simulink model "vco_phase_noise_3"  (Simulink 7.4)
settings: Solver=ode45  StartTime=0.0  StopTime=.01  MaxStep=.4/(100e6)  RelTol=.25e-3
StopFcn:
  | VCO_plot_dbc_per_hz;
values from neighbouring files (symbols this model uses):
  Fs = OverSample*Freq(end)    [VCO_noise_profile_3.m]
undefined symbols (not defined in the file or in its folder): dBc, dfilt, Hz
libraries: dspstat3 x6, dsparch4 x5, simulink x3, dspbuff3 x3, dspsigops x3, dspsnks4 x3, dspspect3 x1, dspsrcs4 x1
settings Model: Creator=dbenson  LastModifiedBy=Dick
settings OptimizationCC: InlineInvariantSignals=on  InitFltsAndDblsToZero=on
settings DebuggingCC: SaveWithParameterizedLinksMsg=none  SignalResolutionControl=TryResolveAllWithWarning  MultiTaskDSMMsg=warning  MultiTaskCondExecSysMsg=none  Int32ToFloatConvMsg=none  StrictBusMsg=None
settings RTWCC: IncludeERTFirstTime=on
settings GRTTargetCC: TargetFcnLib=ansi_tfl_tmw.mat

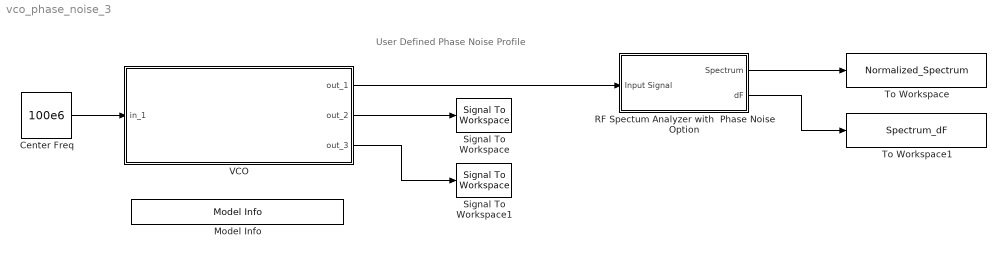
== system vco_phase_noise_3 ==
  note: User Defined Phase Noise Profile
  Center Freq : Constant  Value=100e6  VectorParams1D=off  OutDataType=sfix(16)  OutScaling=2^0
  Model Info : simulink/Model-Wide Utilities/Model Info  SystemSampleTime=-1  InitialBlockCM=None  BlockCM=None  Frame=on  DisplayStringWithTags=Copywrite 2010 The MathWorks, Inc.  HorizontalTextAlignment=Center  LeftAlignmentValue=0.5  SourceBlockDiagram=vco_phase_noise_3  TagMaxNumber=20
  RF Spectum Analyzer with  Phase Noise Option : Subsystem  Description=Spectrum Analyzer  mask{BW=20e6, Fc=100e6, Frame=2^11, Navg=50, N_Toss=2}
      mask prompts: BW "Bandwidth"; Fc "Center Freq"; Frame "Frame Size  (power of 2)"; Navg "Number of Averages"; N_Toss "Toss N Frames b4 Averaging"
      mask Display: fprintf('Spectrum Analyzer \n Fc=%7.2f MHz \n BW=%7.2f MHz',Fc/1e6,BW/1e6)
  Signal To Workspace : dspsnks4/Signal To Workspace  SystemSampleTime=-1  VariableName=Fvec  FrameMode=Concatenate frames (2-D array)
      settings: MaxDataPoints=1  FixptAsFi=off
  Signal To Workspace1 : dspsnks4/Signal To Workspace  SystemSampleTime=-1  VariableName=Lvec  FrameMode=Concatenate frames (2-D array)
      settings: MaxDataPoints=1  FixptAsFi=off
  To Workspace : ToWorkspace  VariableName=Normalized_Spectrum  SampleTime=-1  SaveFormat=Array
      settings: MaxDataPoints=1
  To Workspace1 : ToWorkspace  VariableName=Spectrum_dF  SampleTime=-1  SaveFormat=Array
      settings: MaxDataPoints=1
  VCO : Subsystem  mask{Freq=[ 1e5, 5e5,    2e6,    5e6 ,    8e6   10e6], Level=[-90,   -90,    -100,   -100,    -120 , -120 ]-10, Npts=2^10, OverSample=2.5, Interp_Select=Log X, Ph=0, Kc=1, Fc=0, Ac=sqrt(2)}
      mask prompts: Freq "Phase Noise Freq Vector in Hz"; Level "Phase Noise Level Vector dBc/Hz"; Npts "Phase Noise FIR Filter Length (power of 2)"; OverSample "Phase Noise Oversample (>2)"; Interp_Select "Phase Noise X axis Interpolation"; Ph "Initial Phase (rad)"; Kc "Input Sensitivity (Hz/Volt)"; Fc "Oscillation freq (Hz)"; Ac "Output amplitude (Volt)"
      mask init:
      | Verify=1;
      | noise_filt=VCO_noise_profile_3(Npts,Level,Freq,OverSample,Interp_Select,Verify); 
      | % Npts = length of filter kernel. More provides increased freq resolution
      | % Freq     = Vector of frequencies in Hz
      | % Level = Corresponding Vector of noise levels
      | % Verify   = true to show plots
      | % Create a filter kernel (FIR coefficients) that approximates a user spec'd
      | % power spectrum Level is dB/Hz
      mask StyleString: edit,edit,edit,edit,popup(Linear X|Log X),edit,edit,edit,edit
      mask Display:
      | disp('VCO \nWith User Defined \n Phase Noise (rab)')
      | port_label('input',1','Freq');
      | port_label('output',1','VCO Out');
      | port_label('output',2','Fvec');
      | port_label('output',3','Level');
  wires:
  VCO/1(out_1) -> RF Spectum Analyzer with  Phase Noise Option/1(Input Signal)
  Center Freq/1 -> VCO/1(in_1)
  VCO/2(out_2) -> Signal To Workspace/1
  VCO/3(out_3) -> Signal To Workspace1/1
  RF Spectum Analyzer with  Phase Noise Option/1(Spectrum) -> To Workspace/1
  RF Spectum Analyzer with  Phase Noise Option/2(dF) -> To Workspace1/1

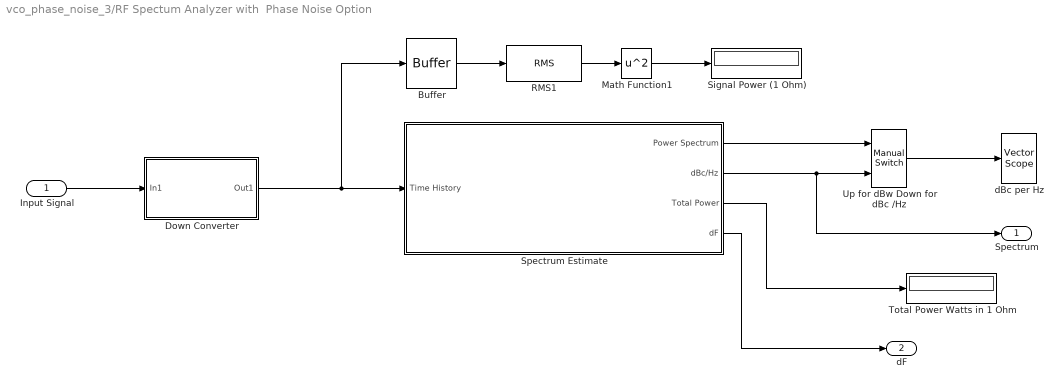
== system vco_phase_noise_3/RF Spectum Analyzer with  Phase Noise Option ==
  Input Signal : Inport  OutDataType=sfix(16)  OutScaling=2^0
  Buffer : dspbuff3/Buffer  N=1024  V=0  ic=0
  Down Converter : Subsystem
  Math Function1 : Math  Operator=square  OutDataType=sfix(16)  OutScaling=2^0  SaturateOnIntegerOverflow=on
  RMS1 : dspstat3/RMS  DialogController=dspDDGCreate  DialogControllerArgs=DataTag0  run=off  reset_popup=None  directionMode=Each column  dimension=1  treatSBRowAsCol=on
  Signal Power (1 Ohm) : Display
  Spectrum Estimate : Subsystem  mask{Frame=Frame, Navg=Navg, N_Toss=N_Toss}
      mask prompts: Frame "Frame Size"; N_Toss "Toos N Frames b4 Averaging"
      mask Display:
      | disp('Power Spectrum \nEstimate')
      | port_label('input',1,'y(t)');
      | port_label('output',1,'Power Spectrum')
      | port_label('output',2,'Scaled for dBc/Hz')
      | port_label('output',3','Total Power');
      | port_label('output',4','dF');
  Total Power Watts in 1 Ohm : Display
  Up for dBw Down for dBc /Hz : simulink/Signal Routing/Manual Switch  SystemSampleTime=-1  sw=0  action=0  varsize=off
  dBc per Hz : dspsnks4/Vector Scope  DialogController=dspdialog.VectorScope  DialogControllerArgs=DataTag5  ScopeProperties=on  Domain=Frequency  HorizSpan=1  DisplayProperties=off  AxisGrid=on  Memory=off  FrameNumber=on  AxisLegend=off  AxisZoom=off  OpenScopeAtSimStart=on  OpenScopeImmediately=off  FigPos=[586 199 560 252]  AxisProperties=off  XUnits=Hertz  XRange=[-Fs/2...Fs/2]  InheritXIncr=on  XIncr=1  XLabel=Time  XLimit=Auto  XMin=0  XMax=1  XStart=0  YUnits=dB  YLabel=dBc/Hz  LineProperties=off  XAxisParamsVer=6.9
      settings: YMin=-164.362362670898  YMax=2.17442076291263e-006
  Spectrum : Outport  OutDataType=fixdt(1, 16)  OutScaling=2^0
  dF : Outport  Port=2  OutDataType=fixdt(1, 16)  OutScaling=2^0
  wires:
  Up for dBw Down for dBc /Hz/1 -> dBc per Hz/1
  Spectrum Estimate/3(Total Power) -> Total Power Watts in 1 Ohm/1
  Spectrum Estimate/2(dBc/Hz) -> Up for dBw Down for dBc /Hz/2, Spectrum/1
  Spectrum Estimate/1(Power Spectrum) -> Up for dBw Down for dBc /Hz/1
  RMS1/1 -> Math Function1/1
  Buffer/1 -> RMS1/1
  Math Function1/1 -> Signal Power (1 Ohm)/1
  Input Signal/1 -> Down Converter/1(In1)
  Down Converter/1(Out1) -> Spectrum Estimate/1(Time History), Buffer/1
  Spectrum Estimate/4(dF) -> dF/1

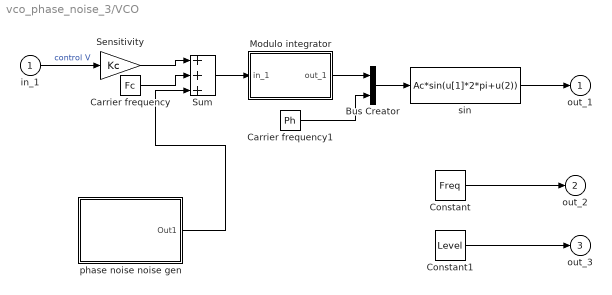
== system vco_phase_noise_3/VCO ==
  in_1 : Inport  OutDataType=sfix(16)  OutScaling=2^0
  Bus Creator : BusCreator  Inputs=2
  Carrier frequency : Constant  Value=Fc  OutDataType=sfix(16)  OutScaling=2^0
  Carrier frequency1 : Constant  Value=Ph  OutDataType=sfix(16)  OutScaling=2^0
  Constant : Constant  Value=Freq  OutDataType=fixdt(1, 16)  OutScaling=2^0
  Constant1 : Constant  Value=Level  OutDataType=fixdt(1, 16)  OutScaling=2^0
  Modulo integrator : Subsystem  mask(Modulo integrator){modu=1, init=0}
      mask prompts: modu "Modulo bound:"; init "Initial state:"
      mask help: When the absolute value of the state exceeds the modulo bound, the state is reset to be the remainder of the state divided by the modulo bound.
      mask Help: This block calculate the integration of the input signal. The absolute value of this integrator will not exceed the specified module bound. The state value is reset to be the remainder of the state divided by the modulo bound. This block can only be used for scale value calculation. This block is a continuous-time integration block.
      mask Display: disp('Modulo\nintegrator')
  Sensitivity : Gain  Gain=Kc  ParameterDataType=sfix(16)  ParameterScaling=2^0  OutDataType=sfix(16)  OutScaling=2^0  SaturateOnIntegerOverflow=on  OutDataTypeStr=Inherit: Same as input  ParamDataTypeStr=Inherit: Same as input
  Sum : Sum  Inputs=+++  OutDataType=sfix(16)  OutScaling=2^0  SaturateOnIntegerOverflow=on  InputSameDT=on  OutDataTypeStr=Inherit: Same as first input
  phase noise noise gen : Subsystem  TreatAsAtomicUnit=on
  sin : Fcn  Expr=Ac*sin(u[1]*2*pi+u(2))
  out_1 : Outport  OutDataType=sfix(16)  OutScaling=2^0
  out_2 : Outport  Port=2  OutDataType=sfix(16)  OutScaling=2^0
  out_3 : Outport  Port=3  OutDataType=sfix(16)  OutScaling=2^0
  wires:
  Modulo integrator/1(out_1) -> Bus Creator/1
  Bus Creator/1 -> sin/1
  Sum/1 -> Modulo integrator/1(in_1)
  sin/1 -> out_1/1
  Carrier frequency/1 -> Sum/2
  Sensitivity/1 -> Sum/1
  in_1/1 -> Sensitivity/1  "control V"
  phase noise noise gen/1(Out1) -> Sum/3
  Constant/1 -> out_2/1
  Constant1/1 -> out_3/1
  Carrier frequency1/1 -> Bus Creator/2

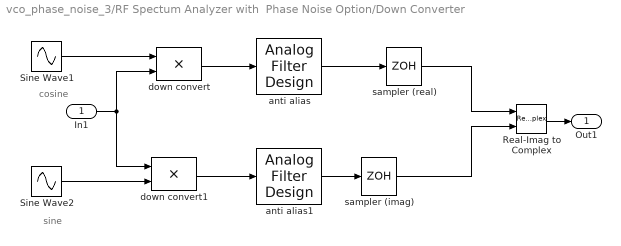
== system vco_phase_noise_3/RF Spectum Analyzer with  Phase Noise Option/Down Converter ==
  note: cosine
  note: sine
  In1 : Inport
  Real-Imag to Complex : RealImagToComplex
  Sine Wave1 : Sin  Amplitude=sqrt(2)  Bias=0  Frequency=2*pi*(Fc)  Phase=-pi/2  Samples=10  SampleTime=0  Offset=0
  Sine Wave2 : Sin  Amplitude=sqrt(2)  Bias=0  Frequency=2*pi*(Fc)  Phase=0  Samples=10  SampleTime=0  Offset=0
  anti alias : dsparch4/Analog Filter Design  method=Elliptic  filttype=Lowpass  N=9  Wlo=BW*pi  Whi=80  Rp=1.2  Rs=100
  anti alias1 : dsparch4/Analog Filter Design  method=Elliptic  filttype=Lowpass  N=9  Wlo=BW*pi  Whi=80  Rp=1.2  Rs=100
  down convert : Product  OutDataType=sfix(16)  OutScaling=2^0  SaturateOnIntegerOverflow=on  InputSameDT=on  OutDataTypeStr=Inherit: Same as first input
  down convert1 : Product  OutDataType=sfix(16)  OutScaling=2^0  SaturateOnIntegerOverflow=on  InputSameDT=on  OutDataTypeStr=Inherit: Same as first input
  sampler (imag) : ZeroOrderHold  SampleTime=1/(1.28*BW)
  sampler (real) : ZeroOrderHold  SampleTime=1/(1.28*BW)
  Out1 : Outport
  wires:
  In1/1 -> down convert/2, down convert1/1
  down convert/1 -> anti alias/1
  anti alias/1 -> sampler (real)/1
  Sine Wave1/1 -> down convert/1
  Sine Wave2/1 -> down convert1/2
  anti alias1/1 -> sampler (imag)/1
  down convert1/1 -> anti alias1/1
  sampler (real)/1 -> Real-Imag to Complex/1
  sampler (imag)/1 -> Real-Imag to Complex/2
  Real-Imag to Complex/1 -> Out1/1

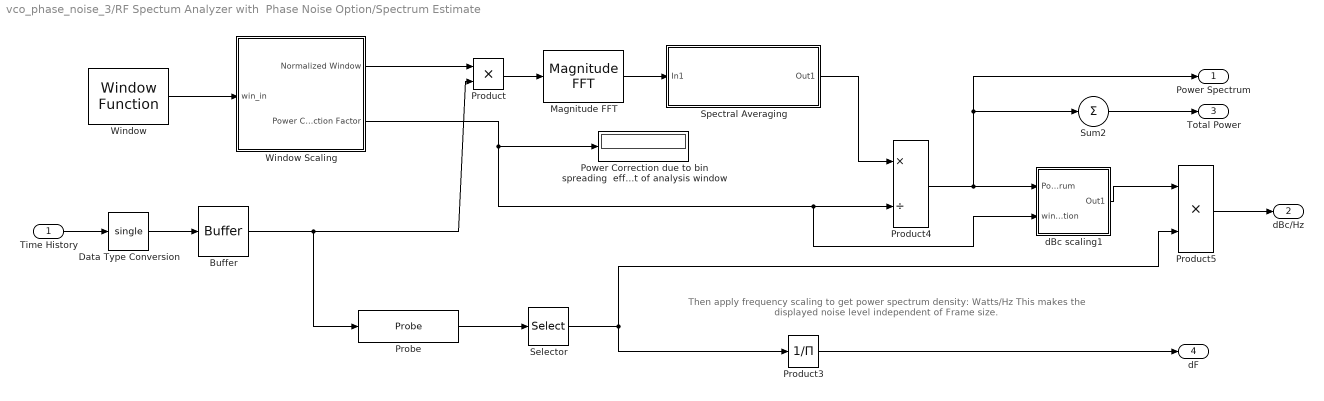
== system vco_phase_noise_3/RF Spectum Analyzer with  Phase Noise Option/Spectrum Estimate ==
  note: Then apply frequency scaling to get power spectrum density: Watts/Hz
      | This makes the displayed noise level independent of Frame size.
  Time History : Inport  OutDataType=sfix(16)  OutScaling=2^0
  Buffer : dspbuff3/Buffer  N=Frame  V=0  ic=0
  Data Type Conversion : DataTypeConversion  OutDataTypeMode=single  OutDataType=sfix(16)  OutScaling=2^0  OutDataTypeStr=single
  Magnitude FFT : dspspect3/Magnitude FFT  SystemSampleTime=-1  mag_or_magsq=Magnitude squared  fftLenInherit=on  fftsize=fftsize
  "Power Correction due to bin spreading  effect of analysis window " : Display
      settings: Decimation=100
  Probe : Probe  ProbeWidth=off  ProbeComplexSignal=off  ProbeWidthDataType=single  ProbeSampleTimeDataType=single
  Product : Product  OutDataType=sfix(16)  OutScaling=2^0  RndMeth=Zero
  Product3 : Product  Inputs=/  OutDataType=sfix(16)  OutScaling=2^0  RndMeth=Zero
  Product4 : Product  Inputs=*/  OutDataType=sfix(16)  OutScaling=2^0  RndMeth=Zero
  Product5 : Product  Inputs=**  OutDataType=sfix(16)  OutScaling=2^0  RndMeth=Zero
  Selector : Selector  InputPortWidth=2  IndexOptions=Index vector (dialog)  Indices=[1]  OutputSizes=1
  Spectral Averaging : Subsystem  mask{Navg=Navg}
      mask Display: disp('Spectral Averaging')
  Sum2 : Sum  Inputs=+  OutDataType=sfix(16)  OutScaling=2^0
  Window : dspsigops/Window Function  DialogController=dspDDGCreate  DialogControllerArgs=DataTag2  winmode=Generate window  wintype=Hanning  sampmode=Discrete  samptime=-1  N=Frame  Rs=60  beta=1  winsamp=Periodic  UserWindow=hamming  OptParams=off  UserParams={1.0}  dataType=single  isSigned=on  wordLen=16  udDataType=sfix(16)  fracBitsMode=Best precision  numFracBits=15  roundingMode=Floor  overflowMode=off  numSidelobes=4  sidelobeLevel=-30
      settings: additionalParams=on
  Window Scaling : Subsystem
  dBc scaling1 : Subsystem
  Power Spectrum : Outport  OutDataType=sfix(16)  OutScaling=2^0
  dBc/Hz : Outport  Port=2  OutDataType=sfix(16)  OutScaling=2^0
  Total Power : Outport  Port=3  OutDataType=sfix(16)  OutScaling=2^0
  dF : Outport  Port=4  OutDataType=sfix(16)  OutScaling=2^0
  wires:
  Product/1 -> Magnitude FFT/1
  Window/1 -> Window Scaling/1(win_in)
  Spectral Averaging/1(Out1) -> Product4/1
  Time History/1 -> Data Type Conversion/1
  Probe/1 -> Selector/1
  Selector/1 -> Product3/1, Product5/2
  Data Type Conversion/1 -> Buffer/1
  Buffer/1 -> Product/2, Probe/1
  Window Scaling/1(Normalized Window) -> Product/1
  Window Scaling/2(Power Correction Factor) -> "Power Correction due to bin spreading  effect of analysis window "/1, Product4/2, dBc scaling1/2(window correction)
  Product3/1 -> dF/1
  Magnitude FFT/1 -> Spectral Averaging/1(In1)
  Product4/1 -> dBc scaling1/1(Power Spectrum), Sum2/1, Power Spectrum/1
  dBc scaling1/1(Out1) -> Product5/1
  Product5/1 -> dBc/Hz/1
  Sum2/1 -> Total Power/1

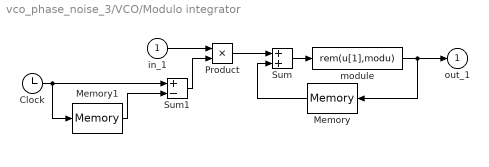
== system vco_phase_noise_3/VCO/Modulo integrator ==
  in_1 : Inport  OutDataType=sfix(16)  OutScaling=2^0
  Clock : Clock
      settings: Decimation=10
  Memory : Memory  X0=init
  Memory1 : Memory
  Product : Product  OutDataType=sfix(16)  OutScaling=2^0  SaturateOnIntegerOverflow=on  InputSameDT=on  OutDataTypeStr=Inherit: Same as first input
  Sum : Sum  OutDataType=sfix(16)  OutScaling=2^0  SaturateOnIntegerOverflow=on  InputSameDT=on  OutDataTypeStr=Inherit: Same as first input
  Sum1 : Sum  Inputs=+-  OutDataType=sfix(16)  OutScaling=2^0  SaturateOnIntegerOverflow=on  InputSameDT=on  OutDataTypeStr=Inherit: Same as first input
  module : Fcn  Expr=rem(u[1],modu)
  out_1 : Outport  OutDataType=sfix(16)  OutScaling=2^0
  wires:
  Memory1/1 -> Sum1/2
  Clock/1 -> Memory1/1, Sum1/1
  in_1/1 -> Product/1
  Sum1/1 -> Product/2
  Memory/1 -> Sum/2
  Product/1 -> Sum/1
  Sum/1 -> module/1
  module/1 -> out_1/1, Memory/1

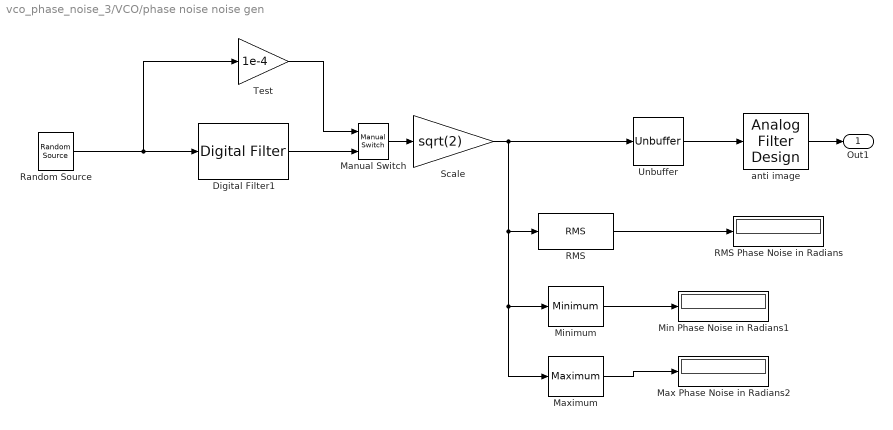
== system vco_phase_noise_3/VCO/phase noise noise gen ==
  Digital Filter1 : dsparch4/Digital Filter  DialogController=dspdialog.DigitalFilter  DialogControllerArgs=DataTag6  TypePopup=FIR (all zeros)  IIRFiltStruct=Direct form II transposed  AllPoleFiltStruct=Direct form  FIRFiltStruct=Direct form  CoeffSource=Specify via dialog  NumCoeffs=noise_filt  DenCoeffs=den  BiQuadCoeffs=[1 0.3 0.4 1 0.1 0.2]  LatticeCoeffs=[0.2 0.4]  denIgnore=on  FiltPerSampPopup=One filter per frame  IC=0  ICnum=0  ICden=0  roundingMode=Floor  overflowMode=off  ScaleValues=1  scaleValueFracLength=14  stageInFracLength=15  stageOutFracLength=15  FilterSource=Specify via dialog  dfiltObjectName=dfilt.dffir([1 2 1])
  Manual Switch : simulink/Signal Routing/Manual Switch  SystemSampleTime=-1  sw=0  action=0  varsize=off
  Max Phase Noise in Radians2 : Display
  Maximum : dspstat3/Maximum  DialogController=dspDDGCreate  DialogControllerArgs=DataTag7  fcn=Value  reset=None  indexBase=One  operateOver=Each column  Dimension=1  colComp=on  operation=maximum  roiEnable=off  roiType=Rectangles  roiPortion=Entire ROI  roiOutput=Individual statistics for each ROI  roiFlag=off  accumDataTypeStr=Inherit: Same as product output  accumLastDataTypeStr=Inherit: Same as product output  roundingMode=Floor  overflowMode=off
  Min Phase Noise in Radians1 : Display
  Minimum : dspstat3/Minimum  DialogController=dspDDGCreate  DialogControllerArgs=DataTag8  fcn=Value  reset=None  indexBase=One  operateOver=Each column  Dimension=1  colComp=on  operation=minimum  roiEnable=off  roiType=Rectangles  roiPortion=Entire ROI  roiOutput=Individual statistics for each ROI  roiFlag=off  roundingMode=Floor  overflowMode=off
  RMS : dspstat3/RMS  DialogController=dspDDGCreate  DialogControllerArgs=DataTag9  run=off  reset_popup=None  directionMode=Each column  dimension=1  treatSBRowAsCol=on
  RMS Phase Noise in Radians : Display
  Random Source : dspsrcs4/Random Source  SrcType=Gaussian  NormMethod=Ziggurat  CltLength=12  MinVal=0  MaxVal=1  MeanVal=0  VarVal=Freq(end)*sqrt(2)  RepMode=Not repeatable  rawSeed=1  IsInherit=off  SampMode=Discrete  SampTime=1/(OverSample*Freq(end))  SampFrame="512  % not critical"  DataType=Double  OutComplex=Real
  "Scale " : Gain  Gain=sqrt(2)  ParameterDataType=fixdt(1, 16)  ParameterScaling=2^0  OutDataType=fixdt(1, 16)  OutScaling=2^0
  Test : Gain  Gain=1e-4  ParameterDataType=fixdt(1, 16)  ParameterScaling=2^0  OutDataType=fixdt(1, 16)  OutScaling=2^0
  Unbuffer : dspbuff3/Unbuffer  ic=0
  anti image : dsparch4/Analog Filter Design  method=Elliptic  filttype=Lowpass  N=8  Wlo=(OverSample/2)*Freq(end)*2*pi  Whi=80  Rp=.5  Rs=100
  Out1 : Outport  OutDataType=sfix(16)  OutScaling=2^0
  wires:
  Random Source/1 -> Digital Filter1/1, Test/1
  anti image/1 -> Out1/1
  Unbuffer/1 -> anti image/1
  RMS/1 -> RMS Phase Noise in Radians/1
  Digital Filter1/1 -> Manual Switch/2
  Manual Switch/1 -> "Scale "/1
  Test/1 -> Manual Switch/1
  Minimum/1 -> Min Phase Noise in Radians1/1
  Maximum/1 -> Max Phase Noise in Radians2/1
  "Scale "/1 -> Unbuffer/1, RMS/1, Minimum/1, Maximum/1

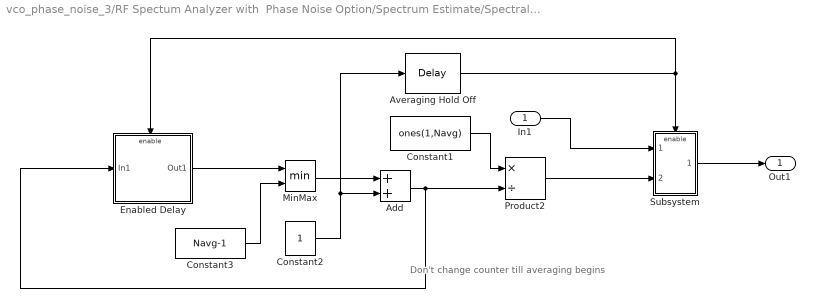
== system vco_phase_noise_3/RF Spectum Analyzer with  Phase Noise Option/Spectrum Estimate/Spectral Averaging ==
  note: Don't change counter
      |  till averaging begins
  In1 : Inport  OutDataType=sfix(16)  OutScaling=2^0
  Add : Sum  OutDataType=sfix(16)  OutScaling=2^-10
  Averaging Hold Off : dspsigops/Delay  dly_unit=Samples  delay=N_Toss  ic_detail=off  dif_ic_for_ch=off  dif_ic_for_dly=off  ic=0  reset_popup=None
  Constant1 : Constant  Value=ones(1,Navg)  OutDataTypeMode=single  OutDataType=sfix(16)  OutScaling=2^0  OutDataTypeStr=single
  Constant2 : Constant  OutDataTypeMode=single  OutDataType=sfix(16)  OutScaling=2^0  OutDataTypeStr=single  SampleTime=Frame/(1.28*BW)
  Constant3 : Constant  Value=Navg-1  OutDataTypeMode=single  OutDataType=sfix(16)  OutScaling=2^0  OutDataTypeStr=single  SampleTime=Frame/(1.28*BW)
  Enabled Delay : Subsystem
  MinMax : MinMax  Inputs=2  OutDataType=sfix(16)  OutScaling=2^0
  Product2 : Product  Inputs=*/  OutDataType=sfix(16)  OutScaling=2^0  RndMeth=Zero
  Subsystem : Subsystem
  Out1 : Outport  OutDataType=sfix(16)  OutScaling=2^0
  wires:
  Add/1 -> Product2/2, Enabled Delay/1(In1)
  Constant2/1 -> Add/2, Averaging Hold Off/1
  Product2/1 -> Subsystem/2(In2)
  Enabled Delay/1(Out1) -> MinMax/1
  MinMax/1 -> Add/1
  Constant3/1 -> MinMax/2
  In1/1 -> Subsystem/1(In1)
  Subsystem/1(Out1) -> Out1/1
  Constant1/1 -> Product2/1
  Averaging Hold Off/1 -> Subsystem/Enable, Enabled Delay/Enable

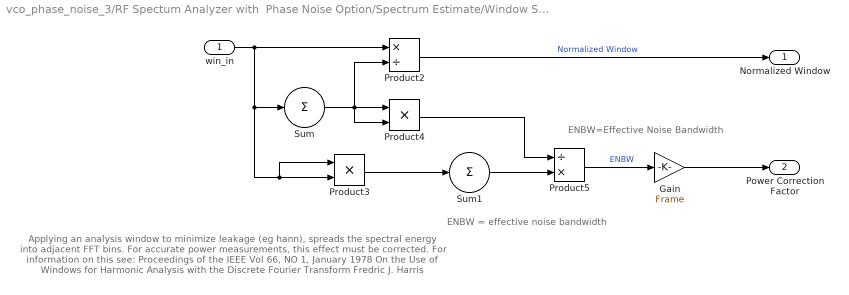
== system vco_phase_noise_3/RF Spectum Analyzer with  Phase Noise Option/Spectrum Estimate/Window Scaling ==
  note: ENBW = effective noise bandwidth
  note: Applying an analysis window to minimize leakage (eg hann),
      | spreads the spectral energy into adjacent FFT bins.
      | For accurate power measurements, this effect must be corrected.
      | For information on this see:
      | Proceedings of the IEEE Vol 66, NO 1, January 1978
      | On the Use of Windows for Harmonic Analysis with the Discrete Fourier Transform
      | Fredric J. Harris
  note: ENBW=Effective Noise Bandwidth
  win_in : Inport  OutDataType=sfix(16)  OutScaling=2^0
  Gain : Gain  Gain=Frame  ParameterDataType=sfix(16)  ParameterScaling=2^0  OutDataType=sfix(16)  OutScaling=2^0
  Product2 : Product  Inputs=*/  OutDataType=sfix(16)  OutScaling=2^0  RndMeth=Zero
  Product3 : Product  OutDataType=sfix(16)  OutScaling=2^0  RndMeth=Zero
  Product4 : Product  OutDataType=sfix(16)  OutScaling=2^0  RndMeth=Zero
  Product5 : Product  Inputs=/*  OutDataType=sfix(16)  OutScaling=2^0  RndMeth=Zero
  Sum : Sum  Inputs=+  OutDataType=sfix(16)  OutScaling=2^0
  Sum1 : Sum  Inputs=+  OutDataType=sfix(16)  OutScaling=2^0
  Normalized Window : Outport  OutDataType=sfix(16)  OutScaling=2^0
  Power Correction Factor : Outport  Port=2  OutDataType=sfix(16)  OutScaling=2^0
  wires:
  Product2/1 -> Normalized Window/1  "Normalized Window"
  Product3/1 -> Sum1/1
  Product4/1 -> Product5/1
  Sum1/1 -> Product5/2
  Product5/1 -> Gain/1  "ENBW"
  win_in/1 -> Sum/1, Product3/1, Product3/2, Product2/1
  Sum/1 -> Product4/1, Product4/2, Product2/2
  Gain/1 -> Power Correction Factor/1

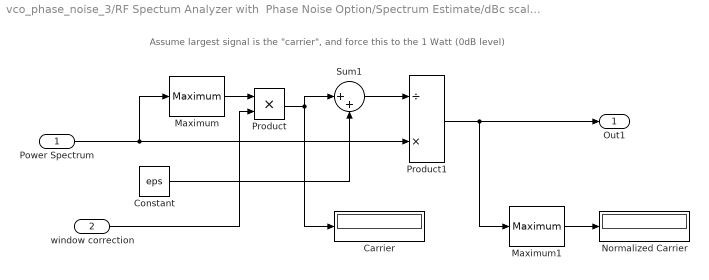
== system vco_phase_noise_3/RF Spectum Analyzer with  Phase Noise Option/Spectrum Estimate/dBc scaling1 ==
  note: Assume largest signal is the "carrier", and force this to the 1 Watt (0dB level)
  Power Spectrum : Inport  OutDataType=sfix(16)  OutScaling=2^0
  window correction : Inport  Port=2  OutDataType=sfix(16)  OutScaling=2^0
  Carrier : Display
  Constant : Constant  Value=eps  OutDataType=sfix(16)  OutScaling=2^0
  Maximum : dspstat3/Maximum  DialogController=dspDDGCreate  DialogControllerArgs=DataTag3  fcn=Value  reset=None  indexBase=One  operateOver=Each column  Dimension=1  colComp=on  operation=maximum  roiEnable=off  roiType=Rectangles  roiPortion=Entire ROI  roiOutput=Individual statistics for each ROI  roiFlag=off  accumDataTypeStr=Inherit: Same as product output  accumLastDataTypeStr=Inherit: Same as product output  roundingMode=Floor  overflowMode=off
  Maximum1 : dspstat3/Maximum  DialogController=dspDDGCreate  DialogControllerArgs=DataTag4  fcn=Value  reset=None  indexBase=One  operateOver=Each column  Dimension=1  colComp=on  operation=maximum  roiEnable=off  roiType=Rectangles  roiPortion=Entire ROI  roiOutput=Individual statistics for each ROI  roiFlag=off  accumDataTypeStr=Inherit: Same as product output  accumLastDataTypeStr=Inherit: Same as product output  roundingMode=Floor  overflowMode=off
  "Normalized Carrier " : Display
  Product : Product  OutDataType=fixdt(1, 16)  OutScaling=2^0  RndMeth=Zero
  Product1 : Product  Inputs=/*  OutDataType=sfix(16)  OutScaling=2^0  RndMeth=Zero
  Sum1 : Sum  Inputs=|++  OutDataType=sfix(16)  OutScaling=2^0
  Out1 : Outport  OutDataType=sfix(16)  OutScaling=2^0
  wires:
  Constant/1 -> Sum1/2
  Sum1/1 -> Product1/1
  Product1/1 -> Out1/1, Maximum1/1
  Power Spectrum/1 -> Product1/2, Maximum/1
  Maximum1/1 -> "Normalized Carrier "/1
  Maximum/1 -> Product/1
  Product/1 -> Sum1/1, Carrier/1
  window correction/1 -> Product/2

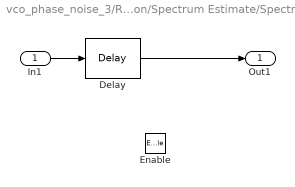
== system vco_phase_noise_3/RF Spectum Analyzer with  Phase Noise Option/Spectrum Estimate/Spectral Averaging/Enabled Delay ==
  In1 : Inport
  Enable : EnablePort
  Delay : dspsigops/Delay  dly_unit=Samples  delay=1  ic_detail=off  dif_ic_for_ch=off  dif_ic_for_dly=off  ic=0  reset_popup=None
  Out1 : Outport
  wires:
  In1/1 -> Delay/1
  Delay/1 -> Out1/1

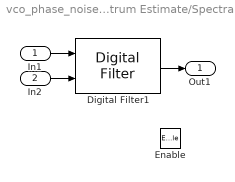
== system vco_phase_noise_3/RF Spectum Analyzer with  Phase Noise Option/Spectrum Estimate/Spectral Averaging/Subsystem ==
  In1 : Inport
  In2 : Inport  Port=2
  Enable : EnablePort
  Digital Filter1 : dsparch4/Digital Filter  DialogController=dspdialog.DigitalFilter  DialogControllerArgs=DataTag1  TypePopup=FIR (all zeros)  IIRFiltStruct=Direct form II transposed  AllPoleFiltStruct=Direct form  FIRFiltStruct=Direct form  CoeffSource=Input port(s)  NumCoeffs=[1 2]  DenCoeffs=[1 0.1]  BiQuadCoeffs=[1 0.3 0.4 1 0.1 0.2]  LatticeCoeffs=[0.2 0.4]  denIgnore=on  FiltPerSampPopup=One filter per frame  IC=0  ICnum=0  ICden=0  roundingMode=Floor  overflowMode=off  ScaleValues=1  scaleValueFracLength=14  stageInFracLength=15  stageOutFracLength=15  FilterSource=Input port(s)  dfiltObjectName=dfilt.dffir([1 2 1])
  Out1 : Outport
  wires:
  In1/1 -> Digital Filter1/1
  Digital Filter1/1 -> Out1/1
  In2/1 -> Digital Filter1/2
